simulink model "Dynamics_TranslationalEoM_TH"  (Simulink 7.9)
settings: Solver=ode45  StartTime=0.0  StopTime=time_span  FixedStep=0.1  MaxStep=10  RelTol=1e-10
values from neighbouring files (symbols this model uses):
  Input_Mass = 500    [Dynamics_TranslationalEoM_Test.m]
undefined symbols (not defined in the file or in its folder): Dynamics, Global
libraries: AeroSim x2
settings Model: Creator=Ryan  LastModifiedBy=ryan
settings GRTTargetCC: CombineOutputUpdateFcns=off  GRTInterface=on

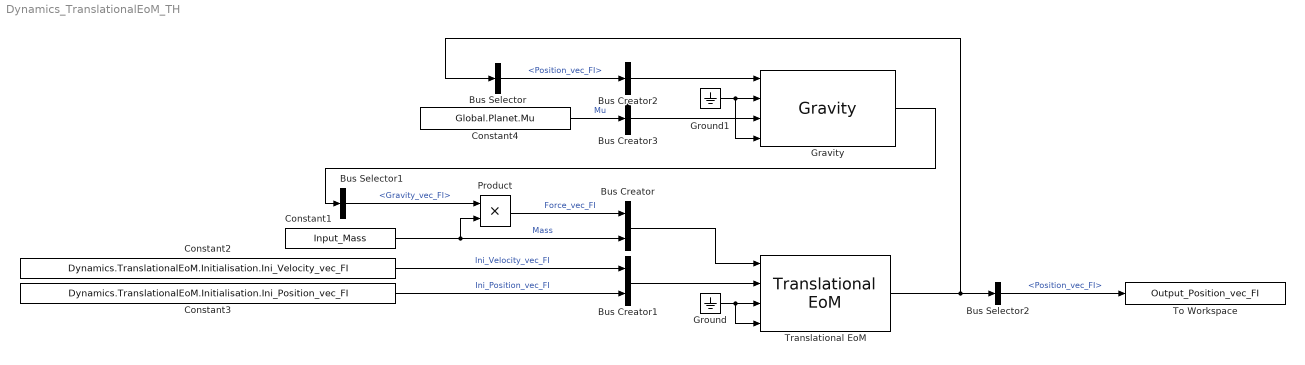
== system Dynamics_TranslationalEoM_TH ==
  Bus Creator : BusCreator  Inputs=2
  Bus Creator1 : BusCreator  Inputs=2
  Bus Creator2 : BusCreator  Inputs=1
  Bus Creator3 : BusCreator  Inputs=1
  Bus Selector : BusSelector  OutputSignals=Position_vec_FI
  Bus Selector1 : BusSelector  OutputSignals=Gravity_vec_FI
  Bus Selector2 : BusSelector  OutputSignals=Position_vec_FI
  Constant1 : Constant  Value=Input_Mass
  Constant2 : Constant  Value=Dynamics.TranslationalEoM.Initialisation.Ini_Velocity_vec_FI
  Constant3 : Constant  Value=Dynamics.TranslationalEoM.Initialisation.Ini_Position_vec_FI
  Constant4 : Constant  Value=Global.Planet.Mu
  Gravity : AeroSim/Environment/Gravity
  Ground : Ground
  Ground1 : Ground
  Product : Product  RndMeth=Zero
  To Workspace : ToWorkspace  VariableName=Output_Position_vec_FI  SampleTime=-1
  Translational EoM : AeroSim/Dynamics/Translational EoM
  wires:
  Ground/1 -> Translational EoM/4, Translational EoM/3
  Constant1/1 -> Bus Creator/2, Product/2  "Mass"
  Product/1 -> Bus Creator/1  "Force_vec_FI"
  Bus Creator/1 -> Translational EoM/1
  Constant3/1 -> Bus Creator1/2  "Ini_Position_vec_FI"
  Constant2/1 -> Bus Creator1/1  "Ini_Velocity_vec_FI"
  Bus Creator1/1 -> Translational EoM/2
  Bus Creator2/1 -> Gravity/1
  Bus Creator3/1 -> Gravity/3
  Ground1/1 -> Gravity/2, Gravity/4
  Constant4/1 -> Bus Creator3/1  "Mu"
  Translational EoM/1 -> Bus Selector/1, Bus Selector2/1
  Bus Selector/1 -> Bus Creator2/1  "<Position_vec_FI>"
  Gravity/1 -> Bus Selector1/1
  Bus Selector1/1 -> Product/1  "<Gravity_vec_FI>"
  Bus Selector2/1 -> To Workspace/1  "<Position_vec_FI>"
